simulink model "mdlref_heater"  (Simulink 6.0)
settings: Solver=ode3  SolverMode=SingleTasking  StartTime=0.0  StopTime=2*24*60*60  FixedStep=60  RelTol=1e-3  AbsTol=1e-6
undefined symbols (not defined in the file or in its folder): ha, Mdot
settings Model: Creator=The MathWorks Inc.  LastModifiedBy=batserve  ExtModeAutoUpdateStatusClock=off
settings DataIOCC: ExternalInput=[]  InitialState=[]  LimitDataPoints=off  SaveOutput=off  SaveTime=off
settings OptimizationCC: BlockReduction=off  BooleanDataType=off  InlineParams=on
settings DebuggingCC: CheckExecutionContextPreStartOutputMsg=on  CheckExecutionContextRuntimeOutputMsg=on  SignalResolutionControl=UseLocalSettings  SolverPrmCheckMsg=none  IntegerOverflowMsg=none
settings HardwareCC: TargetUnknown=on

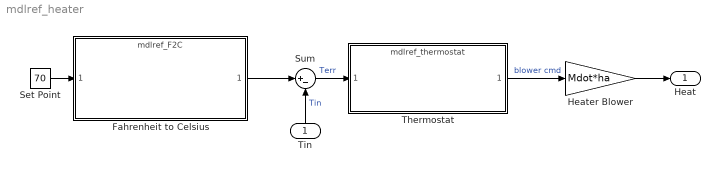
== system mdlref_heater ==
  Tin : Inport  Orientation=up  Port=1  PortDimensions=1  SampleTime=0  DataType=double  LatchInput=off
  Fahrenheit to Celsius : ModelReference  ModelName=mdlref_F2C  ModelReferenceVersion=1.8  CopyOfModelName=mdlref_F2C
  Heater Blower : Gain  Gain=Mdot*ha  SaturateOnIntegerOverflow=on
  Set Point : Constant  Value=70
  Sum : Sum  Inputs=|+-  SaturateOnIntegerOverflow=on  InputSameDT=on
  Thermostat : ModelReference  ModelName=mdlref_thermostat  ModelReferenceVersion=1.8  CopyOfModelName=mdlref_thermostat
  Heat : Outport
  wires:
  Heater Blower/1 -> Heat/1
  Thermostat/1 -> Heater Blower/1  "blower cmd"
  Tin/1 -> Sum/2  "Tin"
  Sum/1 -> Thermostat/1  "Terr"
  Fahrenheit to Celsius/1 -> Sum/1
  Set Point/1 -> Fahrenheit to Celsius/1
